simulink model "EX1_kwa"  (R2023b)
settings: Solver=FixedStepDiscrete  StartTime=0.0  StopTime=0  RelTol=1e-3
libraries: CPOiS_SourcesSinks x10, CPOiS_DataManipulation x6
settings Model: Creator=alyskawa  LastModifiedBy=alyskawa

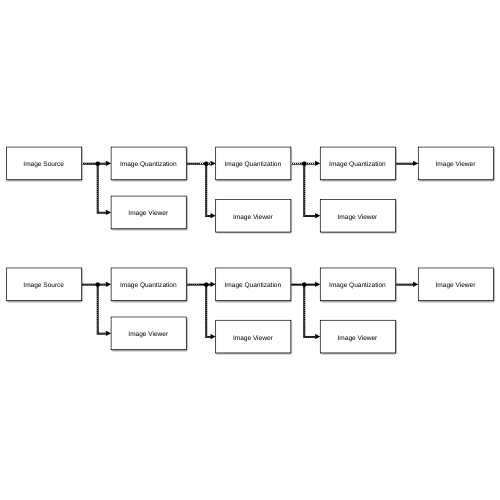
[thumbnail: Simulink's stored preview of the top-level diagram]
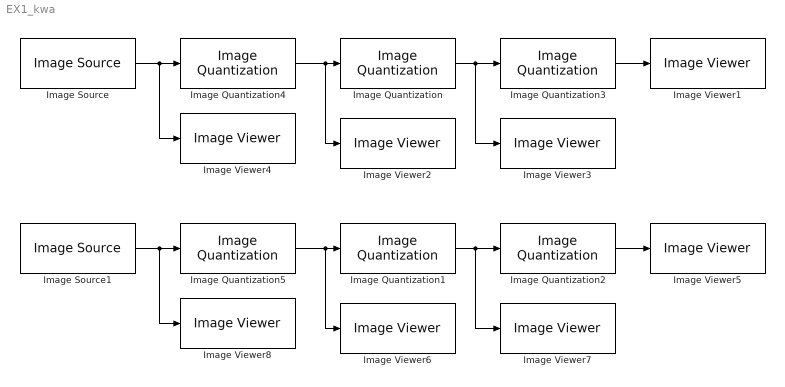
== system EX1_kwa ==
  Image Quantization : CPOiS_DataManipulation/Image Quantization  LevelsNum=8
      settings: SourceProductName=CPOiS - Digital image and signal processing
  Image Quantization1 : CPOiS_DataManipulation/Image Quantization  LevelsNum=8
      settings: SourceProductName=CPOiS - Digital image and signal processing
  Image Quantization2 : CPOiS_DataManipulation/Image Quantization  LevelsNum=12
      settings: SourceProductName=CPOiS - Digital image and signal processing
  Image Quantization3 : CPOiS_DataManipulation/Image Quantization  LevelsNum=12
      settings: SourceProductName=CPOiS - Digital image and signal processing
  Image Quantization4 : CPOiS_DataManipulation/Image Quantization  LevelsNum=4
      settings: SourceProductName=CPOiS - Digital image and signal processing
  Image Quantization5 : CPOiS_DataManipulation/Image Quantization  LevelsNum=4
      settings: SourceProductName=CPOiS - Digital image and signal processing
  Image Source : CPOiS_SourcesSinks/Image Source  FileSelection=ball.png
      settings: SourceProductName=CPOiS - Digital image and signal processing
  Image Source1 : CPOiS_SourcesSinks/Image Source  FileSelection=airport.png
      settings: SourceProductName=CPOiS - Digital image and signal processing
  Image Viewer{1..8} (8 alike) : CPOiS_SourcesSinks/Image Viewer
      settings: SourceProductName=CPOiS - Digital image and signal processing
  wires:
  Image Source/1 -> Image Quantization4/1, Image Viewer4/1
  Image Quantization4/1 -> Image Quantization/1, Image Viewer2/1
  Image Quantization/1 -> Image Quantization3/1, Image Viewer3/1
  Image Quantization3/1 -> Image Viewer1/1
  Image Quantization1/1 -> Image Quantization2/1, Image Viewer7/1
  Image Source1/1 -> Image Quantization5/1, Image Viewer8/1
  Image Quantization5/1 -> Image Quantization1/1, Image Viewer6/1
  Image Quantization2/1 -> Image Viewer5/1
